simulink model "video_grab"  (R2016b)
settings: Solver=VariableStepAuto  StartTime=0.0  StopTime=10  RelTol=1e-3
undefined symbols (not defined in the file or in its folder): none, videoinput
libraries: dspvision x1, imaqlib x1
settings Model: Creator=Thomas  LastModifiedBy=Thomas

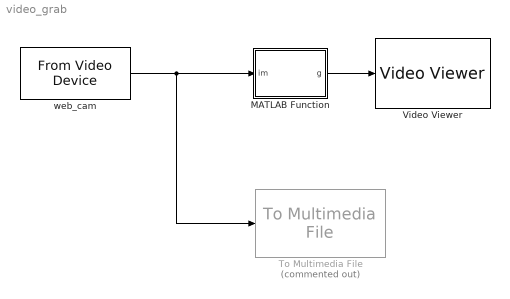
== system video_grab ==
  MATLAB Function : MATLAB Function  TreatAsAtomicUnit=on
  To Multimedia File : dspvision/To Multimedia File  Commented=on  outputFilename=output.avi  streamSelection=Video only  videoCompressor=None (uncompressed)  audioCompressor=None (uncompressed)  imagePorts=One multidimensional signal  fileType=AVI  audioDatatype=Determine from input data type  fourcc=RGB  videoQuality=75  mj2000CompFactor=10
  Video Viewer : VideoViewer  FigPos=[687.4 588.4 409.6 300]
  web_cam : imaqlib/From Video Device  DeviceMenu=winvideo 1 (Integrated Camera)  Device=winvideo 1 (Integrated Camera)  ObjConstructor=videoinput('winvideo', 1)  VideoFormatMenu=YUY2_640x480  VideoFormat=YUY2_640x480  VideoSource=input1  ROIPosition=[0 0 480 640]  EnableHWTrigger=off  TriggerConfiguration=none/none  SampleTime=1/30  OutputPortsMode=One multidimensional signal  DataType=single  CanDoHWTrigger=no  ReturnedColorSpace=rgb  BlockHandle=6.0001  ROIWidth=640  ROIHeight=480  ROIColumn=0  ROIRow=0  EngXMLPath=C:\Program Files\MATLAB\R2016b\toolbox\imaq\imaq\private  DevXMLPath=C:\ProgramData\MATLAB\SupportPackages\R2016b\toolbox\imaq\supportpackages\genericvideo\adaptor\win64  EngLibPath=C:\Program Files\MATLAB\R2016b\toolbox\imaq\imaqblks\imaqmex\win64  ColorSpace=rgb  BayerSensorAlignment=grbg
  wires:
  web_cam/1 -> MATLAB Function/1(im), To Multimedia File/1
  MATLAB Function/1(g) -> Video Viewer/1

== matlab function video_grab/MATLAB Function ==
  data: im input; g output
function g = fcn(im)

    %im = vid.grab;
    %if isempty(im), break; end
    %im = iroi(im,roi);
    [ilg ihg] = size(im);
    %% RGB to HSI
    R=im(:,:,1);
    G=im(:,:,2);
    B=im(:,:,3);
     %Hue
    numi=1/2*((R-G)+(R-B));
    denom=((R-G).^2+((R-B).*(G-B))).^0.5;
    %To avoid divide by zero exception add a small number in the denominator
    H=acosd(numi./(denom+0.000001));
    %If B>G then H= 360-Theta
    H(B>G)=360-H(B>G);
    %Normalize to the range [0 1]
    H=H/360;
    %Saturation
    S=1- (3./(sum(im,3)+0.000001)).*min(im,[],3);
    %Intensity
    I=sum(im,3)./3;
    im = ((0.8)*im(:,:,1)+0.1*im(:,:,2)+0.1*im(:,:,3));    
     %HSI
    HSI=zeros([480 640 3]);
    HSI(:,:,1)=H;
    HSI(:,:,2)=S;
    HSI(:,:,3)=I;
    g = zeros(size(H));
    %% Treshholding 
    for i = 1:640
       for j = 1:480
       if (H(i,j) >= 0.5 && H(i,j) <= 0.66 && S(i,j) >= 0.4 && S(i,j) <= 1)
           g(i,j) = 1;
       else 
           g(i,j) = 0;
       end
       end
    end
